simulink model "Ex2_5_2_6"  (R2016a)
settings: Solver=VariableStepAuto  StartTime=0.0  StopTime=10.0  RelTol=1e-3
settings Model: Creator=mende  LastModifiedBy=mende

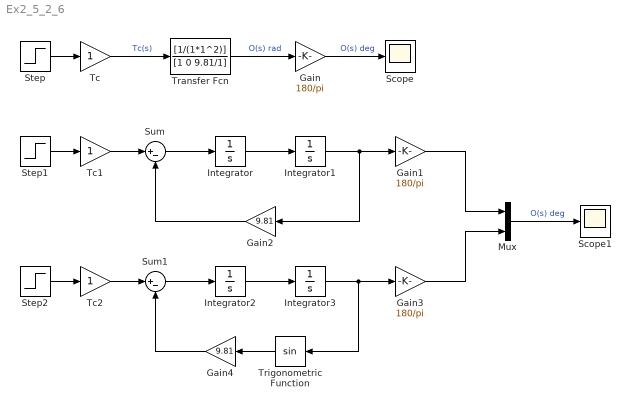
== system Ex2_5_2_6 ==
  Gain : Gain  Gain=180/pi
  Gain1 : Gain  Gain=180/pi
  Gain2 : Gain  Gain=9.81
  Gain3 : Gain  Gain=180/pi
  Gain4 : Gain  Gain=9.81
  Integrator{,1..3} (4 alike) : Integrator
  Mux : Mux  Inputs=2
  Scope : Scope
  Scope1 : Scope
  Step : Step  Time=0  SampleTime=0
  Step1 : Step  Time=0  SampleTime=0
  Step2 : Step  Time=0  SampleTime=0
  Sum : Sum  Inputs=|+-
  Sum1 : Sum  Inputs=|+-
  Tc : Gain
  Tc1 : Gain
  Tc2 : Gain
  Transfer Fcn : TransferFcn  Numerator=[1/(1*1^2)]  Denominator=[1 0 9.81/1]
  Trigonometric Function : Trigonometry
  wires:
  Transfer Fcn/1 -> Gain/1  "O(s) rad"
  Gain/1 -> Scope/1  "O(s) deg"
  Step1/1 -> Tc1/1
  Tc1/1 -> Sum/1
  Sum/1 -> Integrator/1
  Integrator/1 -> Integrator1/1
  Integrator1/1 -> Gain2/1, Gain1/1
  Gain2/1 -> Sum/2
  Step2/1 -> Tc2/1
  Tc2/1 -> Sum1/1
  Sum1/1 -> Integrator2/1
  Integrator2/1 -> Integrator3/1
  Integrator3/1 -> Trigonometric Function/1, Gain3/1
  Gain4/1 -> Sum1/2
  Trigonometric Function/1 -> Gain4/1
  Mux/1 -> Scope1/1  "O(s) deg"
  Gain3/1 -> Mux/2
  Gain1/1 -> Mux/1
  Tc/1 -> Transfer Fcn/1  "Tc(s)"
  Step/1 -> Tc/1
